simulink model "pathGeometry_th"  (R2018b)
settings: Solver=FixedStepAuto  StartTime=0.0  StopTime=10.0  FixedStep=.001  RelTol=1e-3
libraries: pathGeometry_ul x1
settings Model: Creator=mcobb  LastModifiedBy=jldanie5

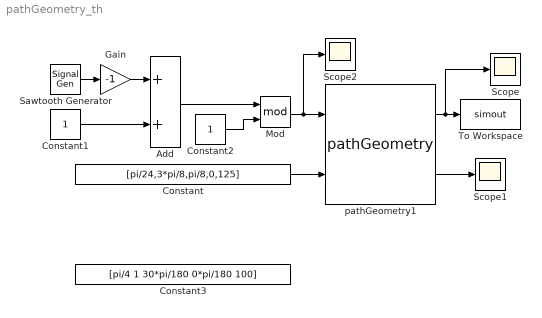
== system pathGeometry_th ==
  Add : Sum
  Constant : Constant  Value=[pi/24,3*pi/8,pi/8,0,125]
  Constant1 : Constant
  Constant2 : Constant
  Constant3 : Constant  Value=[pi/4 1 30*pi/180 0*pi/180 100]
  Gain : Gain  Gain=-1
  Mod : Math  Operator=mod  SaturateOnIntegerOverflow=on
  Sawtooth Generator : SignalGenerator  WaveForm=sawtooth  Amplitude=0.5  Units=rad/sec
  Scope : Scope
  Scope1 : Scope
  Scope2 : Scope
  To Workspace : ToWorkspace  VariableName=simout  SaveFormat=Timeseries  SampleTime=-1
  pathGeometry1 : pathGeometry_ul/pathGeometry  SystemSampleTime=-1
  wires:
  pathGeometry1/1 -> Scope/1, To Workspace/1
  Constant1/1 -> Add/2
  Mod/1 -> Scope2/1, pathGeometry1/1
  Add/1 -> Mod/1
  Constant2/1 -> Mod/2
  pathGeometry1/2 -> Scope1/1
  Sawtooth Generator/1 -> Gain/1
  Gain/1 -> Add/1
  Constant/1 -> pathGeometry1/2
